simulink model "lineControl"  (R2018b)
settings: Solver=VariableStepAuto  StartTime=0.0  StopTime=5  FixedStep=Ts  RelTol=1e-3
InitFcn:
  | lCScript
values from neighbouring files (symbols this model uses):
  A = [1 0; Ts*vt 1]    [lCScript.m]
  B = [Ts; 0]    [lCScript.m]
  C = [0 1]    [lCScript.m]
  K = acker(A, B, phic)    [lCScript.m]
  maxvr = 1.82    [lCScript.m]
  Ts = 1/60    (= 0.0166666666667)    [lCScript.m]
  vt = 0.22    [lCScript.m]
  x0 = [pi/2; 0]    [lCScript.m]
libraries: simulink x1
settings Model: Creator=User  LastModifiedBy=User

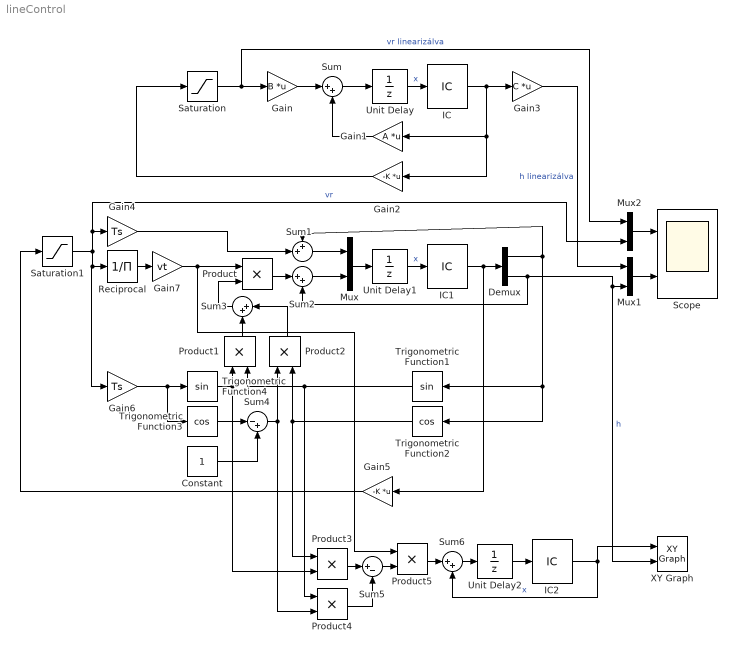
== system lineControl ==
  Constant : Constant
  Demux : Demux  Outputs=2
  Gain : Gain  Gain=B  Multiplication=Matrix(K*u)
  Gain1 : Gain  Gain=A  Multiplication=Matrix(K*u)
  Gain2 : Gain  Gain=-K  Multiplication=Matrix(K*u)
  Gain3 : Gain  Gain=C  Multiplication=Matrix(K*u)
  Gain4 : Gain  Gain=Ts
  Gain5 : Gain  Gain=-K  Multiplication=Matrix(K*u)
  Gain6 : Gain  Gain=Ts
  Gain7 : Gain  Gain=vt
  IC : InitialCondition  Value=x0
  IC1 : InitialCondition  Value=x0
  IC2 : InitialCondition  Value=0
  Mux : Mux  Inputs=2
  Mux1 : Mux  Inputs=2
  Mux2 : Mux  Inputs=2
  Product{,1..5} (6 alike) : Product
  Reciprocal : Product  Inputs=/
  Saturation : Saturate  UpperLimit=maxvr  LowerLimit=-maxvr
  Saturation1 : Saturate  UpperLimit=maxvr  LowerLimit=-maxvr
  Scope : Scope  NumInputPorts=2
  Sum{,2..3,6} (4 alike) : Sum  Inputs=|++
  Sum1 : Sum  Inputs=++|
  Sum4 : Sum  Inputs=|-+
  Sum5 : Sum  Inputs=|+-
  Trigonometric Function1 : Trigonometry
  Trigonometric Function2 : Trigonometry  Operator=cos
  Trigonometric Function3 : Trigonometry  Operator=cos
  Trigonometric Function4 : Trigonometry
  Unit Delay : UnitDelay  SampleTime=Ts
  Unit Delay1 : UnitDelay  SampleTime=Ts
  Unit Delay2 : UnitDelay  SampleTime=Ts
  XY Graph : simulink/Sinks/XY Graph  xmin=0  xmax=1  ymin=-0.2  ymax=0.2  st=Ts
  wires:
  Sum/1 -> Unit Delay/1
  Gain/1 -> Sum/1
  Gain1/1 -> Sum/2
  Gain2/1 -> Saturation/1
  Unit Delay/1 -> IC/1  "x"
  IC/1 -> Gain2/1, Gain1/1, Gain3/1
  Saturation/1 -> Mux2/1, Gain/1  "vr linearizálva"
  Mux2/1 -> Scope/1
  Mux1/1 -> Scope/2
  Gain3/1 -> Mux1/1  "h linearizálva"
  IC1/1 -> Gain5/1, Demux/1
  Unit Delay1/1 -> IC1/1  "x"
  Mux/1 -> Unit Delay1/1
  Demux/2 -> Sum2/2, XY Graph/2, Mux1/2  "h"
  Saturation1/1 -> Gain6/1, Reciprocal/1, Mux2/2, Gain4/1  "vr"
  Sum1/1 -> Mux/1
  Sum2/1 -> Mux/2
  Gain4/1 -> Sum1/2
  Demux/1 -> Sum1/1, Trigonometric Function2/1, Trigonometric Function1/1
  Gain5/1 -> Saturation1/1
  Reciprocal/1 -> Gain7/1
  Product/1 -> Sum2/1
  Sum3/1 -> Product/2
  Gain7/1 -> Product5/1, Product/1
  Product1/1 -> Sum3/2
  Gain6/1 -> Trigonometric Function4/1, Trigonometric Function3/1
  Trigonometric Function4/1 -> Product3/2, Product1/1
  Trigonometric Function3/1 -> Sum4/1
  Constant/1 -> Sum4/2
  Sum4/1 -> Product2/1, Product4/2
  Trigonometric Function2/1 -> Product3/1, Product2/2
  Product2/1 -> Sum3/1
  Unit Delay2/1 -> IC2/1
  IC2/1 -> Sum6/2, XY Graph/1  "x"
  Trigonometric Function1/1 -> Product4/1, Product1/2
  Sum6/1 -> Unit Delay2/1
  Product5/1 -> Sum6/1
  Product3/1 -> Sum5/1
  Product4/1 -> Sum5/2
  Sum5/1 -> Product5/2
